simulink model "Simulink_Accel"  (R2015a)
settings: Solver=ode4  StartTime=0.0  StopTime=10.0  FixedStep=.01  RelTol=1e-3
model workspace (MATLAB code in the model file):
  | load test3.mat
  | %  geometry = StructHullGeometry('Cedarville');
  | m.InitialValue = 'geometry.m';
  | L.InitialValue = 'geometry.L';
  | LCG.InitialValue = 'geometry.LCG';
  | VCG.InitialValue = 'geometry.VCG';
  | b.InitialValue = 'geometry.b';
  | beta.InitialValue = 'geometry.beta';
  | a.InitialValue = 'geometry.a';
  | f.InitialValue = 'geometry.f';
  | epsilon.InitialValue = 'geometry.epsilon';
  | g.InitialValue = 'physics.g';
  | rho.InitialValue = 'physics.rho';
  | % clear geometry
  | % C = eval('geometry.m')
values from neighbouring files (symbols this model uses):
  intervalle_tau = [1 12]    [Savitsky1964_statique_input_power.m]    (also in Savitsky1964_statique_input_power_old.m; test_tiberlot.m)
  N = (m*g + Df*sind(tau)-T*sind(tau+epsilon))/cosd(tau)    [statique_input_vitesse.m]
  T = sqrt((Df*cos(tau)+N*sin(tau))^2+(m*g-N*cos(tau)+Df*sin(tau))^2)    [CalculSymbolique.m]    (also in statique_input_vitesse.m = (m*g*sind(tau)+Df)/cosd(epsilon))
undefined symbols (not defined in the file or in its folder): v0x
settings Model: Creator=charl  LastModifiedBy=charl

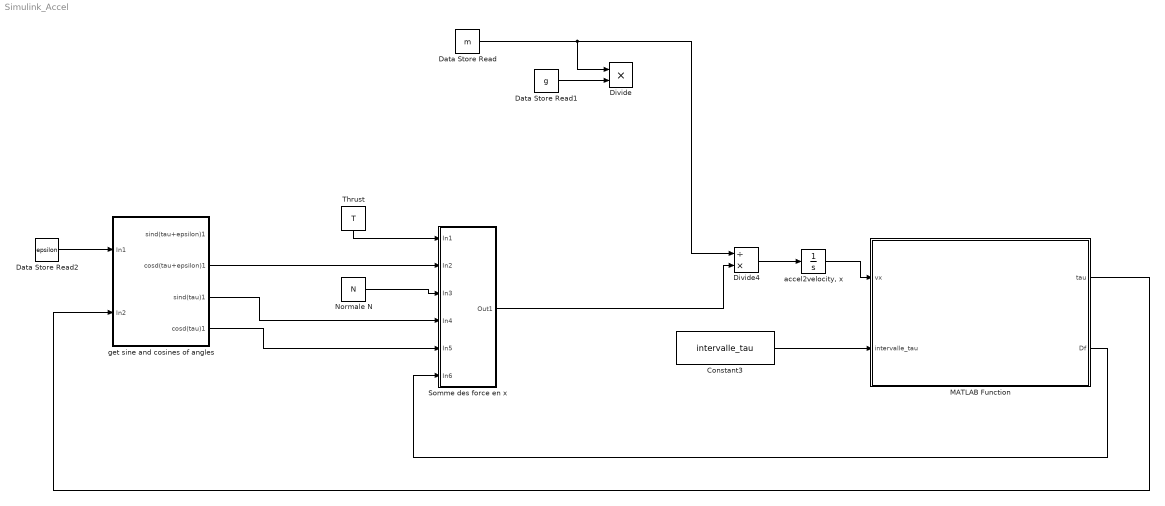
== system Simulink_Accel ==
  Constant3 : Constant  Value=intervalle_tau  VectorParams1D=off
  Data Store Read : DataStoreRead  DataStoreName=m
  Data Store Read1 : DataStoreRead  DataStoreName=g
  Data Store Read2 : DataStoreRead  DataStoreName=epsilon
  Divide : Product  Inputs=**
  Divide4 : Product  Inputs=/*
  MATLAB Function : MATLAB Function  TreatAsAtomicUnit=on
  Normale N : Constant  Value=N
  Somme des force en x : Subsystem
  Thrust : Constant  Value=T
  "accel2velocity, x" : Integrator  InitialCondition=v0x
  get sine and cosines of angles : Subsystem
  wires:
  Data Store Read/1 -> Divide4/1, Divide/1
  Data Store Read2/1 -> get sine and cosines of angles/1(In1)
  Divide4/1 -> "accel2velocity, x"/1
  Thrust/1 -> Somme des force en x/1(In1)
  get sine and cosines of angles/2(cosd(tau+epsilon)1) -> Somme des force en x/2(In2)
  Normale N/1 -> Somme des force en x/3(In3)
  get sine and cosines of angles/3(sind(tau)1) -> Somme des force en x/4(In4)
  get sine and cosines of angles/4(cosd(tau)1) -> Somme des force en x/5(In5)
  Somme des force en x/1(Out1) -> Divide4/2
  "accel2velocity, x"/1 -> MATLAB Function/1(vx)
  MATLAB Function/1(tau) -> get sine and cosines of angles/2(In2)
  MATLAB Function/2(Df) -> Somme des force en x/6(In6)
  Constant3/1 -> MATLAB Function/2(intervalle_tau)
  Data Store Read1/1 -> Divide/2

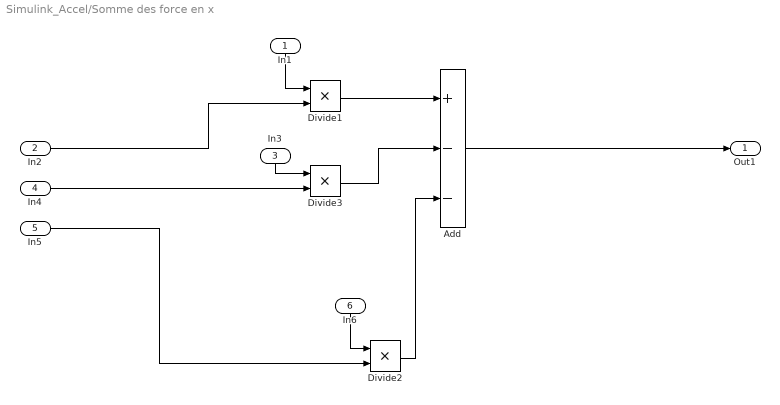
== system Simulink_Accel/Somme des force en x ==
  In1 : Inport
  In2 : Inport  Port=2
  In3 : Inport  Port=3
  In4 : Inport  Port=4
  In5 : Inport  Port=5
  In6 : Inport  Port=6
  Add : Sum  Inputs=+--
  Divide1 : Product  Inputs=**
  Divide2 : Product  Inputs=**
  Divide3 : Product  Inputs=**
  Out1 : Outport
  wires:
  In4/1 -> Divide3/2
  In5/1 -> Divide2/2
  Divide3/1 -> Add/2
  In1/1 -> Divide1/1
  In6/1 -> Divide2/1
  Divide1/1 -> Add/1
  In3/1 -> Divide3/1
  Divide2/1 -> Add/3
  Add/1 -> Out1/1
  In2/1 -> Divide1/2

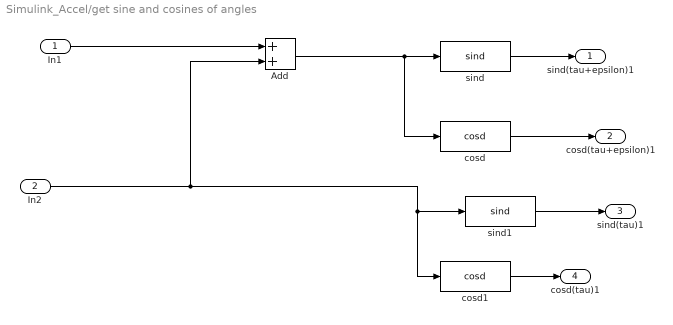
== system Simulink_Accel/get sine and cosines of angles ==
  In1 : Inport
  In2 : Inport  Port=2
  Add : Sum
  cosd : MATLABFcn  MATLABFcn=cosd
  cosd1 : MATLABFcn  MATLABFcn=cosd
  sind : MATLABFcn  MATLABFcn=sind
  sind1 : MATLABFcn  MATLABFcn=sind
  sind(tau+epsilon)1 : Outport
  cosd(tau+epsilon)1 : Outport  Port=2
  sind(tau)1 : Outport  Port=3
  cosd(tau)1 : Outport  Port=4
  wires:
  In1/1 -> Add/1
  Add/1 -> cosd/1, sind/1
  In2/1 -> Add/2, cosd1/1, sind1/1
  sind/1 -> sind(tau+epsilon)1/1
  cosd/1 -> cosd(tau+epsilon)1/1
  sind1/1 -> sind(tau)1/1
  cosd1/1 -> cosd(tau)1/1

== matlab function Simulink_Accel/MATLAB Function ==
  data: vx input size=1; tau output size=1; intervalle_tau input size=2; Df output size=1; m data_store_memory size=1; L data_store_memory size=1; LCG data_store_memory size=1; VCG data_store_memory size=1; b data_store_memory size=1; beta data_store_memory size=1; a data_store_memory size=1; f data_store_memory; epsilon data_store_memory; g data_store_memory; rho data_store_memory
function [tau,Df] = Call_Savitsky1964_statique_input_vitesse_fcn(vx,intervalle_tau)
% fonction pour caller Savitsky1964_statique_input_vitesse_fcn
global g
global rho
global m L LCG VCG b beta a f epsilon

[tau,~,~,Df] = Savitsky1964_statique_input_vitesse_fcn(vx,intervalle_tau);
%%
%% Ajouter les variables globales
% GlobalHullGeometry('SavitskyExample'); % load hull geometry
% GlobalHullGeometry('Cedarville');
% global m L LCG VCG b beta a f epsilon
% global g
% g = 9.81;% m/s2, accélération gravitationnelle
% global rho
% rho = 1000; % kg/m3; eau douce = 1000; eau salée = 1025
% Planing coefficients
% Cv = v/sqrt(g*b);
% CL_beta = m*g/(0.5*rho*v^2*b^2);% lift coefficient pour un angle beta.
% Déjà calculés dans la fonction statique_input_vitesse_v2
% Calculs
% [tau, ~,Df] = bissection_fcn_v_input(intervalle_tau(1),intervalle_tau(end),0.001,vx);
% P_e = D_e*v;
